simulink model "Thermal_model_scope"  (R2018b)
settings: Solver=VariableStepDiscrete  StartTime=0.0  StopTime=300  RelTol=1e-3
libraries: powerlib x25
settings Model: Creator=Prabesh  LastModifiedBy=Prabesh

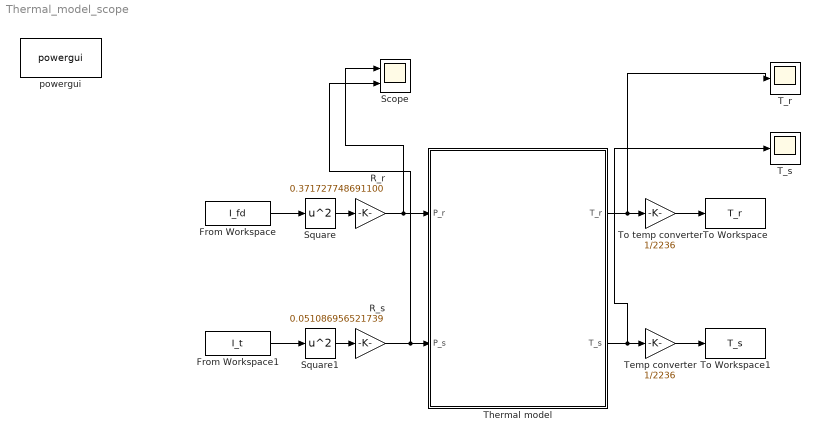
== system Thermal_model_scope ==
  From Workspace : FromWorkspace  VariableName=I_fd  SampleTime=0
  From Workspace1 : FromWorkspace  VariableName=I_t  SampleTime=0
  R_r : Gain  Gain=0.371727748691100
  R_s : Gain  Gain=0.051086956521739
  Scope : Scope  NumInputPorts=2
  Square : Math  Operator=square  SaturateOnIntegerOverflow=on
  Square1 : Math  Operator=square  SaturateOnIntegerOverflow=on
  T_r : Scope
  T_s : Scope
  Temp converter : Gain  Gain=1/2236
  Thermal model : Subsystem
  To Workspace : ToWorkspace  VariableName=T_r  SaveFormat=Timeseries  SampleTime=-1
  To Workspace1 : ToWorkspace  VariableName=T_s  SaveFormat=Timeseries  SampleTime=-1
  To temp converter : Gain  Gain=1/2236
  powergui : powerlib/powergui  Priority=1  SimulationMode=Discrete  SampleTime=300/2402  frequency=60  Iterations=50  frequencyindice=0  Pbase=100e6  ErrMax=1e-4  UnitsV=kV  UnitsW=MW  buscounter=0  FunctionMessages=off  echomessages=off  EnableUseOfTLC=off  CurrentSourceSwitches=off  DisableSnubberDevices=off  DisableRonSwitches=off  DisableVfSwitches=off  DisplayEquations=off  SolverType=Tustin/Backward Euler (TBE)  Interpol=off  ExternalGateDelay=off  methode=off  Ts=100  x0status=blocks  SPID=on  SwTol=0  HookPort=off  RestoreLinks=warning  ResistiveCurrentMeasurement=off  Frange=[0:2:500]  Ylog=off  Xlog=on  ShowGrid=off  save=off  variable=ZData  structure=0  ZoomFFT=off  StartTime=0.0  cycles=1  DisplayStyle=1  fundamental=60  FreqAxis=off  MaxFrequency=1000  frequencyindicesteady=1  RmsSteady=1  display=off
  wires:
  R_r/1 -> Scope/1, Thermal model/1(P_r)
  R_s/1 -> Scope/2, Thermal model/2(P_s)
  Square/1 -> R_r/1
  Square1/1 -> R_s/1
  From Workspace/1 -> Square/1
  From Workspace1/1 -> Square1/1
  Thermal model/1(T_r) -> T_r/1, To temp converter/1
  To temp converter/1 -> To Workspace/1
  Temp converter/1 -> To Workspace1/1
  Thermal model/2(T_s) -> T_s/1, Temp converter/1

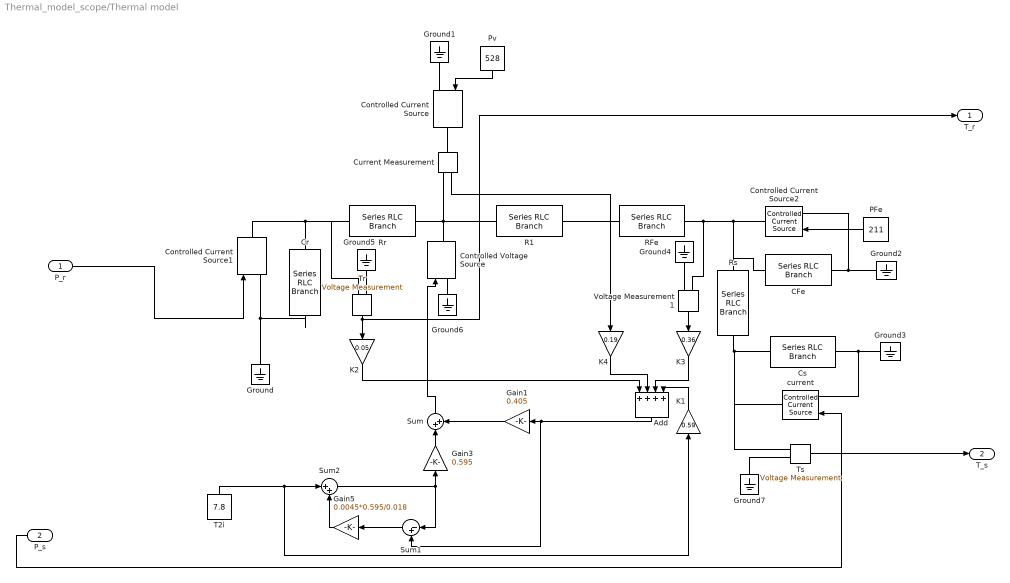
== system Thermal_model_scope/Thermal model ==
  P_r : Inport
  P_s : Inport  Port=2
  Add : Sum  Inputs=++++
  CFe : powerlib/Elements/Series RLC Branch  LConnTagsString=__new0  RConnTagsString=__new0  BranchType=C  Resistance=1  Inductance=1e-3  SetiL0=off  InitialCurrent=0  Capacitance=1.053889273714960e+02  Setx0=off  InitialVoltage=0  Measurements=None
  Controlled Current Source : powerlib/Electrical Sources/Controlled Current Source  Initialize=on  Source_Type=DC  Amplitude=50  Phase=0  Frequency=0  Measurements=None
  Controlled Current Source1 : powerlib/Electrical Sources/Controlled Current Source  Initialize=off  Source_Type=DC  Amplitude=50  Phase=0  Frequency=0  Measurements=None
  Controlled Current Source2 : powerlib/Electrical Sources/Controlled Current Source  Initialize=on  Source_Type=DC  Amplitude=50  Phase=0  Frequency=0  Measurements=None
  Controlled Voltage Source : powerlib/Electrical Sources/Controlled Voltage Source  Initialize=on  Source_Type=AC  Amplitude=0  Phase=0  Frequency=0  Measurements=None
  Cr : powerlib/Elements/Series RLC Branch  LConnTagsString=__new0  RConnTagsString=__new0  BranchType=C  Resistance=1  Inductance=1e-3  SetiL0=off  InitialCurrent=0  Capacitance=11.082786293192750  Setx0=on  InitialVoltage=62636  Measurements=None
  Cs : powerlib/Elements/Series RLC Branch  LConnTagsString=__new0  RConnTagsString=__new0  BranchType=C  Resistance=1  Inductance=1e-3  SetiL0=off  InitialCurrent=0  Capacitance=8.162484073388182  Setx0=on  InitialVoltage=62636  Measurements=None
  Current Measurement : powerlib/Measurements/Current Measurement  PhasorSimulation=off  OutputType=Magnitude  PSBequivalent=0
  Gain1 : Gain  Gain=0.405
  Gain3 : Gain  Gain=0.595
  Gain5 : Gain  Gain=0.0045*0.595/0.018
  Ground{,1..7} (8 alike) : powerlib/Elements/Ground  LConnTagsString=a
  K1 : Gain  Gain=0.59
  K2 : Gain  Gain=0.05
  K3 : Gain  Gain=0.36
  K4 : Gain  Gain=0.19
  PFe : Constant  Value=211
  Pv : Constant  Value=528
  R1 : powerlib/Elements/Series RLC Branch  LConnTagsString=__new0  RConnTagsString=__new0  BranchType=R  Resistance=0.017953321364452  Inductance=1e-3  SetiL0=off  InitialCurrent=0  Capacitance=1e-6  Setx0=off  InitialVoltage=0  Measurements=None
  RFe : powerlib/Elements/Series RLC Branch  LConnTagsString=__new0  RConnTagsString=__new0  BranchType=R  Resistance=0.070224016808497  Inductance=1e-3  SetiL0=off  InitialCurrent=0  Capacitance=1e-6  Setx0=off  InitialVoltage=0  Measurements=None
  Rr : powerlib/Elements/Series RLC Branch  LConnTagsString=__new0  RConnTagsString=__new0  BranchType=R  Resistance=0.371727748691100  Inductance=1e-3  SetiL0=off  InitialCurrent=0  Capacitance=1e-6  Setx0=off  InitialVoltage=0  Measurements=None
  Rs : powerlib/Elements/Series RLC Branch  LConnTagsString=__new0  RConnTagsString=__new0  BranchType=R  Resistance=0.051086956521739  Inductance=1e-3  SetiL0=off  InitialCurrent=0  Capacitance=1e-6  Setx0=off  InitialVoltage=0  Measurements=None
  Sum : Sum  Inputs=|++
  Sum1 : Sum  Inputs=|-+
  Sum2 : Sum  Inputs=|++
  T2i : Constant  Value=7.8
  Tr : powerlib/Measurements/Voltage Measurement  PhasorSimulation=off  OutputType=Magnitude  PSBequivalent=0
  Ts : powerlib/Measurements/Voltage Measurement  PhasorSimulation=off  OutputType=Magnitude  PSBequivalent=0
  Voltage Measurement1 : powerlib/Measurements/Voltage Measurement  PhasorSimulation=off  OutputType=Magnitude  PSBequivalent=0
  current : powerlib/Electrical Sources/Controlled Current Source  Initialize=off  Source_Type=DC  Amplitude=25  Phase=0  Frequency=0  Measurements=None
  T_r : Outport
  T_s : Outport  Port=2
  wires:
  Sum1/1 -> Gain5/1
  Add/1 -> Sum1/2, Gain1/1
  Sum2/1 -> Sum1/1, Gain3/1
  K2/1 -> Add/1
  Ts/1 -> T_s/1
  PFe/1 -> Controlled Current Source2/1
  Gain1/1 -> Sum/2
  T2i/1 -> K1/1, Sum2/1
  K4/1 -> Add/2
  Tr/1 -> T_r/1, K2/1
  K1/1 -> Add/4
  Gain5/1 -> Sum2/2
  K3/1 -> Add/3
  Sum/1 -> Controlled Voltage Source/1
  Voltage Measurement1/1 -> K3/1
  Gain3/1 -> Sum/1
  Current Measurement/1 -> K4/1
  Pv/1 -> Controlled Current Source/1
  P_s/1 -> current/1
  P_r/1 -> Controlled Current Source1/1
  connections:
  Rs/RConn1 -- Ts/LConn1 -- current/RConn1 -- Cs/LConn1
  Ground2/LConn1 -- Controlled Current Source2/LConn1 -- CFe/RConn1
  Ground5/LConn1 -- Tr/LConn2
  Ground4/LConn1 -- Voltage Measurement1/LConn2
  Controlled Current Source2/RConn1 -- CFe/LConn1 -- Rs/LConn1 -- RFe/RConn1 -- Voltage Measurement1/LConn1
  Ground/LConn1 -- Cr/RConn1 -- Controlled Current Source1/LConn1
  Controlled Current Source1/RConn1 -- Tr/LConn1 -- Rr/LConn1 -- Cr/LConn1
  RFe/LConn1 -- R1/RConn1
  R1/LConn1 -- Current Measurement/RConn1 -- Controlled Voltage Source/RConn1 -- Rr/RConn1
  Controlled Current Source/RConn1 -- Current Measurement/LConn1
  Ground6/LConn1 -- Controlled Voltage Source/LConn1
  Ground1/LConn1 -- Controlled Current Source/LConn1
  Ground7/LConn1 -- Ts/LConn2
  Ground3/LConn1 -- current/LConn1 -- Cs/RConn1
